simulink model "furnace_task"  (Simulink 7.5)
libraries: mathlib x34, logiclib x13, analoglib x6, speclib x4, genlib x1
settings Model: Creator=jsobota  LastModifiedBy=jsobota  ExtModeTrigMode=oneshot  ExtModeArmWhenConnect=off

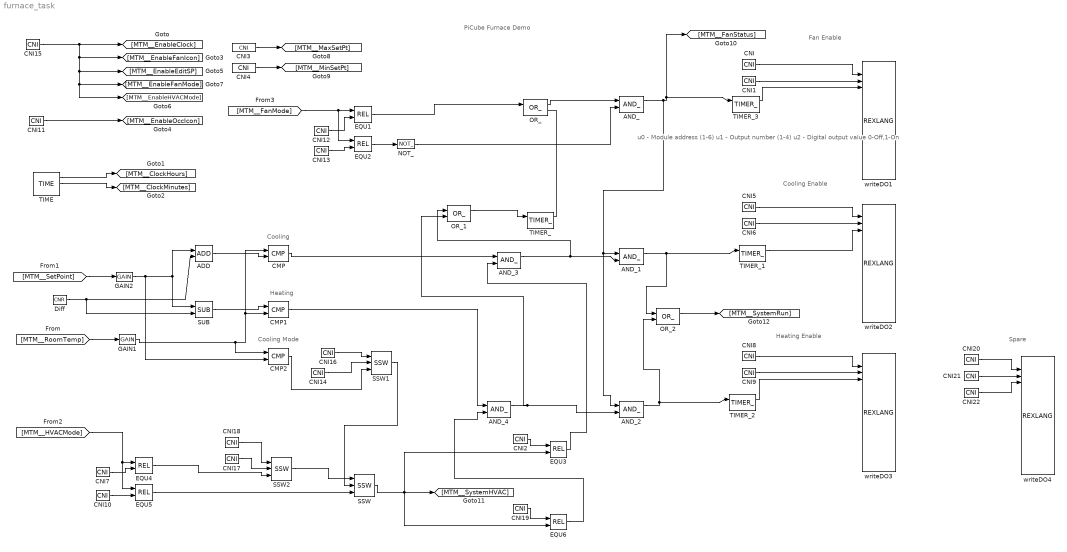
== system furnace_task ==
  note: u0 - Module address (1-6)
      | u1 - Output number (1-4)
      | u2  - Digital output value 0-Off,1-On
  note: PiCube Furnace Demo
  note: Fan Enable
  note: Cooling Enable
  note: Heating Enable
  note: Cooling
  note: Heating
  note: Cooling Mode
  note: Spare
  ADD : mathlib/ADD
  AND_{,1..4} (5 alike) : logiclib/AND_
  CMP : analoglib/CMP  hys=0.50
  CMP1 : analoglib/CMP  hys=0.50
  CMP2 : analoglib/CMP  hys=0.5
  CNI{,1,5,7..8,12,15..17,19..20} (11 alike) : mathlib/CNI  icn=1
  CNI10 : mathlib/CNI  icn=2
  CNI{2,11,13..14,18,22} (6 alike) : mathlib/CNI  icn=0
  CNI21 : mathlib/CNI  icn=4
  CNI3 : mathlib/CNI  icn=280
  CNI4 : mathlib/CNI  icn=180
  CNI6 : mathlib/CNI  icn=2
  CNI9 : mathlib/CNI  icn=3
  Diff : mathlib/CNR  ycn=0.50
  EQU{1..6} (6 alike) : mathlib/REL  irel=1: equality (==)
  GAIN1 : mathlib/GAIN  k=0.1
  GAIN2 : mathlib/GAIN  k=0.1
  NOT_ : logiclib/NOT_
  OR_ : logiclib/OR_
  OR_1 : logiclib/OR_
  OR_2 : logiclib/OR_
  SSW : analoglib/SSW
  SSW1 : analoglib/SSW
  SSW2 : analoglib/SSW
  SUB : mathlib/SUB
  TIME : genlib/TIME  tz=1: Local time
  TIMER_ : logiclib/TIMER_  mode=3: Delayed OFF  pt=30
  TIMER_1 : logiclib/TIMER_  mode=4: Delayed change  pt=5
  TIMER_2 : logiclib/TIMER_  mode=4: Delayed change  pt=5
  TIMER_3 : logiclib/TIMER_  mode=4: Delayed change  pt=5
  writeDO{1..4} (4 alike) : speclib/REXLANG  SystemSampleTime=-1  tab_matlab=BASIC  srcname=writeDO.c  srctype=1: STL  stack=0  debug=1: No check  p0=0  p1=0  p2=0  p3=0  p4=0  p5=0  p6=0  p7=0  p8=0  p9=0  p10=0  p11=0  p12=0  p13=0  p14=0  p15=0  fname=/dev/i2c-1
  wires:
  ADD/1 -> CMP/2
  AND_/1 -> AND_1/1, AND_2/1, [MTM__FanStatus], TIMER_3/1
  AND_1/1 -> OR_2/1, TIMER_1/1
  AND_2/1 -> OR_2/2, TIMER_2/1
  AND_3/1 -> AND_1/2, OR_1/1
  AND_4/1 -> AND_2/2, OR_1/2
  CMP/1 -> AND_3/1
  CMP1/1 -> AND_4/1
  CMP2/1 -> SSW1/3
  CNI/1 -> writeDO1/2
  CNI1/1 -> writeDO1/3
  CNI10/1 -> EQU5/2
  CNI11/1 -> [MTM__EnableOccIcon]
  CNI12/1 -> EQU1/2
  CNI13/1 -> EQU2/2
  CNI14/1 -> SSW1/2
  CNI15/1 -> [MTM__EnableClock], [MTM__EnableFanIcon], [MTM__EnableEditSP], [MTM__EnableHVACMode], [MTM__EnableFanMode]
  CNI16/1 -> SSW1/1
  CNI17/1 -> SSW2/2
  CNI18/1 -> SSW2/1
  CNI19/1 -> EQU6/1
  CNI2/1 -> EQU3/1
  CNI20/1 -> writeDO4/2
  CNI21/1 -> writeDO4/3
  CNI22/1 -> writeDO4/4
  CNI3/1 -> [MTM__MaxSetPt]
  CNI4/1 -> [MTM__MinSetPt]
  CNI5/1 -> writeDO2/2
  CNI6/1 -> writeDO2/3
  CNI7/1 -> EQU4/2
  CNI8/1 -> writeDO3/2
  CNI9/1 -> writeDO3/3
  Diff/1 -> ADD/2, SUB/2
  EQU1/1 -> OR_/1
  EQU2/1 -> NOT_/1
  EQU3/1 -> AND_3/2
  EQU4/1 -> SSW2/3
  EQU5/1 -> SSW/3
  EQU6/1 -> AND_4/2
  [MTM__RoomTemp] -> GAIN1/1
  [MTM__SetPoint] -> GAIN2/1
  [MTM__HVACMode] -> EQU4/1, EQU5/1
  [MTM__FanMode] -> EQU1/1, EQU2/1
  GAIN1/1 -> CMP/1, CMP1/2, CMP2/1
  GAIN2/1 -> CMP2/2, ADD/1, SUB/1
  NOT_/1 -> AND_/2
  OR_/1 -> AND_/1
  OR_1/1 -> TIMER_/1
  OR_2/1 -> [MTM__SystemRun]
  SSW/1 -> EQU3/2, EQU6/2, [MTM__SystemHVAC]
  SSW1/1 -> SSW/2
  SSW2/1 -> SSW/1
  SUB/1 -> CMP1/1
  TIME/1 -> [MTM__ClockHours]
  TIME/2 -> [MTM__ClockMinutes]
  TIMER_/1 -> OR_/2
  TIMER_1/1 -> writeDO2/4
  TIMER_2/1 -> writeDO3/4
  TIMER_3/1 -> writeDO1/4
